simulink model "RLC_Closed_Loop_With_Controller"  (R2019b)
settings: Solver=FixedStepAuto  StartTime=0.0  StopTime=10.0  RelTol=1e-3  EnableMultiTasking=on
undefined symbols (not defined in the file or in its folder): DiscIntNeverNeededParam
libraries: arduinolib x3
settings Model: SILPILModeSetting=veronly  ExtModeTrigDuration=2  Creator=riley  LastModifiedBy=riley
settings OptimizationCC: EnhancedBackFolding=on  PassReuseOutputArgsAs=Individual arguments  ZeroExternalMemoryAtStartup=off  ZeroInternalMemoryAtStartup=off  MaxStackSize=64  OptimizeBlockOrder=speed  DifferentSizesBufferReuse=on  OptimizationCustomize=off  EfficientTunableParamExpr=on
settings DebuggingCC: ParameterPrecisionLossMsg=none  ParameterTunabilityLossMsg=error
settings HardwareCC: ProdBitPerInt=16  ProdBitPerPointer=16  ProdBitPerSizeT=16  ProdBitPerPtrDiffT=16  ProdLargestAtomicFloat=None  ProdWordSize=8  ProdHWDeviceType=Atmel->AVR  UseEmbeddedCoderFeatures=off  UseSimulinkCoderFeatures=off
settings SFSimCC: MATLABDynamicMemAlloc=off
settings RTWCC: SystemTargetFile=ert.tlc  HardwareBoard=Arduino Mega 2560  TLCOptions=-aInlineSetEventsForThisBaseRateFcn=TLC_FALSE -aSuppressMultiTaskScheduler=TLC_FALSE -aRateBasedStepFcn=1  TemplateMakefile=ert_default_tmf  GenerateReport=on  Toolchain=Arduino AVR  BuildConfiguration=Faster Runs  IncludeHyperlinkInReport=on  LaunchReport=on  GenerateTraceInfo=on  GenerateTraceReport=on  GenerateTraceReportSl=on  GenerateTraceReportSf=on  GenerateTraceReportEml=on
settings CodeAppCC: ForceParamTrailComments=on  IgnoreCustomStorageClasses=off  OperatorAnnotations=on  SimulinkDataObjDesc=on  SFDataObjDesc=on  InsertBlockDesc=on
settings ERTTargetCC: SupportContinuousTime=on  SupportNonInlinedSFcns=on  SupportVariableSizeSignals=on  ExtModeStaticAllocSize=2048

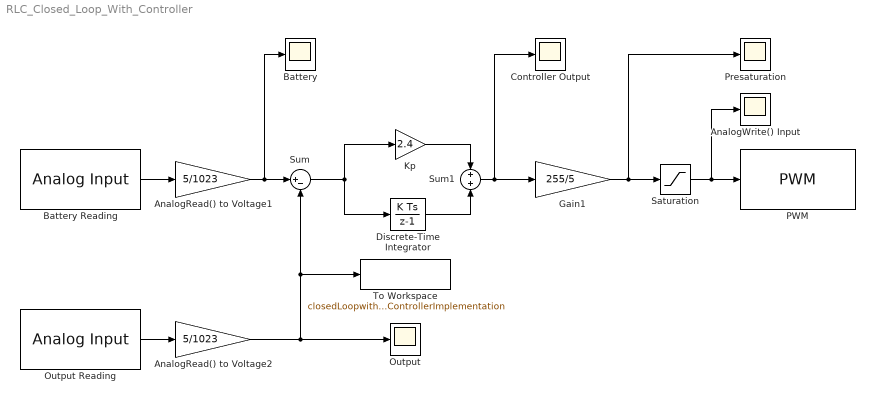
== system RLC_Closed_Loop_With_Controller ==
  "AnalogRead() to Voltage1 " : Gain  Gain=5/1023
  "AnalogRead() to Voltage2 " : Gain  Gain=5/1023
  "AnalogWrite() Input " : Scope
  Battery : Scope
  "Battery Reading " : arduinolib/Analog Input  pinNumber=1  ReadResultsOnly=off  ConversionTriggerSource=Software  ExternalTriggerType=uint32(0)  OutputDataType=uint16  EnableConversionCompleteNotify=off  EnableOuputStatus=off  SampleTime=0.01  blockPlatform=arduino
  "Controller Output " : Scope
  Discrete-Time Integrator : DiscreteIntegrator  gainval=24  SampleTime=0.01  ICPrevOutput=DiscIntNeverNeededParam  ICPrevScaledInput=DiscIntNeverNeededParam
  Gain1 : Gain  Gain=255/5
  Kp : Gain  Gain=2.4
  Output : Scope
  Output Reading : arduinolib/Analog Input  pinNumber=0  ReadResultsOnly=off  ConversionTriggerSource=Software  ExternalTriggerType=uint32(0)  OutputDataType=uint16  EnableConversionCompleteNotify=off  EnableOuputStatus=off  SampleTime=0.01  blockPlatform=arduino
  PWM : arduinolib/PWM  pinNumber=8  EnableInputFrequency=off  InitialFrequency=2000  InitialDutyCycle=0  NotificationType=None  blockPlatform=arduino
  "Presaturation " : Scope
  Saturation : Saturate  UpperLimit=80  LowerLimit=0
  Sum : Sum  Inputs=|+-
  Sum1 : Sum  Inputs=+|+
  To Workspace : ToWorkspace  VariableName=closedLoopwithControllerImplementation  SampleTime=0.01
  wires:
  "Battery Reading "/1 -> "AnalogRead() to Voltage1 "/1
  "AnalogRead() to Voltage2 "/1 -> Sum/2, To Workspace/1, Output/1
  Output Reading/1 -> "AnalogRead() to Voltage2 "/1
  "AnalogRead() to Voltage1 "/1 -> Battery/1, Sum/1
  Kp/1 -> Sum1/1
  Sum/1 -> Discrete-Time Integrator/1, Kp/1
  Sum1/1 -> Gain1/1, "Controller Output "/1
  Discrete-Time Integrator/1 -> Sum1/2
  Gain1/1 -> Saturation/1, "Presaturation "/1
  Saturation/1 -> "AnalogWrite() Input "/1, PWM/1
